simulink model "SistemSortareBandaTransportoare"  (R2025b)
settings: Solver=ode45  StartTime=0.0  StopTime=60  MaxStep=0.01  RelTol=1e-3
libraries: slpidlib x1
settings Model: Creator=Carina  LastModifiedBy=Carina

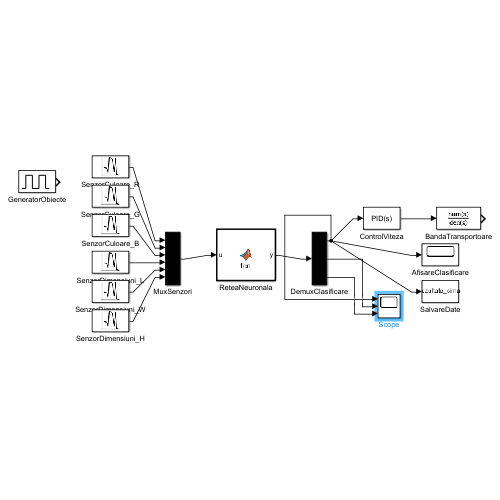
[thumbnail: Simulink's stored preview of the top-level diagram]
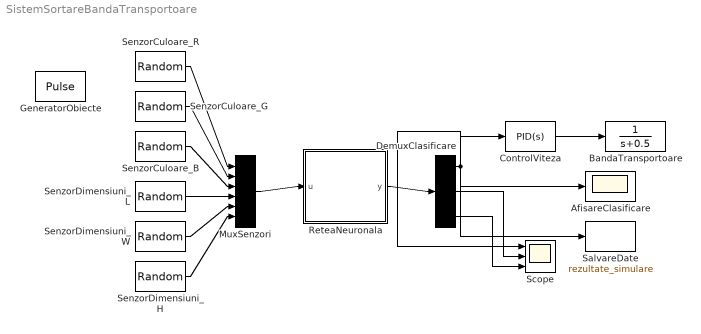
== system SistemSortareBandaTransportoare ==
  AfisareClasificare : Scope
      settings: ActiveDisplayYMinimum=-0.36488795691519493  ActiveDisplayYMaximum=1.6245350457686565
  BandaTransportoare : TransferFcn  Denominator=[1 0.5]
  ControlViteza : slpidlib/PID Controller  Controller=PID  Form=Parallel  TimeDomain=Continuous-time  UseExternalTs=off  SampleTime=-1  IntegratorMethod=Forward Euler  FilterMethod=Forward Euler  ControllerParametersSource=internal  P=1  I=1  UseKiTs=off  D=0  UseExternalDerivativeSource=off  N=100  UseFilter=on  TunerSelectOption=Transfer Function Based (PID Tuner App)  InitialConditionSource=internal  InitialConditionForIntegrator=0  InitialConditionForFilter=0  DifferentiatorICPrevScaledInput=0  ExternalReset=none  TrackingMode=off  Kt=1  LimitOutput=off  SatLimitsSource=internal  UpperSaturationLimit=inf  LowerSaturationLimit=-inf  LinearizeAsGain=on  AntiWindupMode=none  Kb=1  LimitIntegrator=off  UpperIntegratorSaturationLimit=inf  LowerIntegratorSaturationLimit=-inf  POutMin=[]  POutMax=[]  IOutMin=[]  IOutMax=[]  DOutMin=[]  DOutMax=[]  NOutMin=[]  NOutMax=[]  SumOutMin=[]  SumOutMax=[]  SaturationOutMin=[]  SaturationOutMax=[]  PParamMin=[]  PParamMax=[]  IParamMin=[]  IParamMax=[]  DParamMin=[]  DParamMax=[]  NParamMin=[]  NParamMax=[]  KbParamMin=[]  KbParamMax=[]  KtParamMin=[]  KtParamMax=[]  KbOutMin=[]  KbOutMax=[]  KtOutMin=[]  KtOutMax=[]  IntegratorOutMin=[]  IntegratorOutMax=[]  FilterOutMin=[]  FilterOutMax=[]  SumI1OutMin=[]  SumI1OutMax=[]  SumI2OutMin=[]  SumI2OutMax=[]  SumI3OutMin=[]  SumI3OutMax=[]  SumI4OutMin=[]  SumI4OutMax=[]  SumDOutMin=[]  SumDOutMax=[]  DifferentiatorOutMin=[]  DifferentiatorOutMax=[]  FilterDiffOutCoefMin=[]  FilterDiffOutCoefMax=[]  ReciprocalOutMin=[]  ReciprocalOutMax=[]  SumDenOutMin=[]  SumDenOutMax=[]  SumNumOutMin=[]  SumNumOutMax=[]  DivideOutMin=[]  DivideOutMax=[]  UdiffTsProdOutMin=[]  UdiffTsProdOutMax=[]  NTsProdOutMin=[]  NTsProdOutMax=[]  UintegralTsProdOutMin=[]  UintegralTsProdOutMax=[]  UngainTsProdOutMin=[]  UngainTsProdOutMax=[]  ClampingZeroOutDataTypeStr=Inherit: Inherit via back propagation  ClampingZeroOutMin=[]  ClampingZeroOutMax=[]  FilterDenConstantOutDataTypeStr=Inherit: Inherit via back propagation  FilterDenConstantOutMin=[]  FilterDenConstantOutMax=[]  PCopyOutDataTypeStr=Inherit: Inherit via back propagation  PCopyOutMin=[]  PCopyOutMax=[]  NCopyOutDataTypeStr=Inherit: Inherit via back propagation  NCopyOutMin=[]  NCopyOutMax=[]  IntegratorContinuousStateAttributes=''  IntegratorStateMustResolveToSignalObject=off  IntegratorRTWStateStorageClass=Auto  FilterContinuousStateAttributes=''  FilterStateMustResolveToSignalObject=off  FilterRTWStateStorageClass=Auto  ParallelPVariant=InternalParameters  IdealPVariant=Disabled  IVariant=InternalParameters  DVariant=InternalParameters  IntegratorVariant=Continuous  SatVariant=Disabled  AWVariant=Passthrough  PCopyVariant=Disabled  TRVariant=Disabled  FdbkBlocksVariant=Forward  IdealPFdbkVariant=Disabled  SatFdbkVariant=Disabled  DerivativeFilterVariant=ContFilter  NVariant=InternalParameters  NCopyVariant=Disabled  FilterICVariant=InternalICsFilter  IntegratorICVariant=InternalICs  ExternalResetVariant=Disabled  TRSumVariant=Passthrough  SumFdbkVariant=Disabled  SumVariant=Sum_PID  TsampFilterVariant=InternalTs  TsampNgainVariant=Passthrough  TsampIntegralVariant=Disabled_SignalSpec  ExternalSaturationOutDataTypeStr=Inherit: Same as second input  DerivativeSourceVariant=ErrorSignal  PreIntVariant=InternalPreInt
  DemuxClasificare : Demux  Outputs=3
  GeneratorObiecte : DiscretePulseGenerator  PulseType=Time based  PulseWidth=50
  MuxSenzori : Mux  Inputs=6
  ReteaNeuronala : MATLAB Function  TreatAsAtomicUnit=on
  SalvareDate : ToWorkspace  VariableName=rezultate_simulare  SaveFormat=Timeseries  SampleTime=-1
  Scope : Scope  NumInputPorts=3
      settings: ActiveDisplayYMinimum=-0.8870164568392116  ActiveDisplayYMaximum=1.6800836415005935
  SenzorCuloare_B : RandomNumber  Mean=128  Variance=50  SampleTime=0.1
  SenzorCuloare_G : RandomNumber  Mean=128  Variance=50  SampleTime=0.1
  SenzorCuloare_R : RandomNumber  Mean=128  Variance=50  SampleTime=0.1
  SenzorDimensiuni_H : RandomNumber  Mean=0.10  Variance=0.03  SampleTime=0.1
  SenzorDimensiuni_L : RandomNumber  Mean=0.15  Variance=0.05  SampleTime=0.1
  SenzorDimensiuni_W : RandomNumber  Mean=0.15  Variance=0.05  SampleTime=0.1
  wires:
  SenzorCuloare_R/1 -> MuxSenzori/1
  SenzorCuloare_G/1 -> MuxSenzori/2
  SenzorCuloare_B/1 -> MuxSenzori/3
  SenzorDimensiuni_L/1 -> MuxSenzori/4
  SenzorDimensiuni_W/1 -> MuxSenzori/5
  SenzorDimensiuni_H/1 -> MuxSenzori/6
  MuxSenzori/1 -> ReteaNeuronala/1(u)
  ReteaNeuronala/1(y) -> DemuxClasificare/1
  DemuxClasificare/1 -> Scope/1, SalvareDate/1, ControlViteza/1, AfisareClasificare/1
  ControlViteza/1 -> BandaTransportoare/1
  DemuxClasificare/2 -> Scope/2
  DemuxClasificare/3 -> Scope/3

== matlab function SistemSortareBandaTransportoare/ReteaNeuronala ==
  data: u input; y output
function y = fcn(u)
% u = [R G B L W H] (senzorii)
% y = [Plastic; Metal; Sticla] (vector cu 3 ieșiri)

% Normalizare manuală simplă
R = u(1)/255;
G = u(2)/255;
B = u(3)/255;
L = u(4)/0.3;
W = u(5)/0.3;
H = u(6)/0.3;

% Exemplu pseudo-clasificare (logică demo)
plastic_score = 1.5 - abs(R-0.5)*0.5 - L*0.2 - W*0.2;
metal_score   = (R+G+B)/3 + (L+W+H)*0.1;
sticla_score  = 1 - abs(G-0.6)*0.4 + H*0.2;

scores = [plastic_score, metal_score, sticla_score];

% Softmax, întotdeauna vector-coloană
exps = exp(scores - max(scores));
y = (exps ./ sum(exps))';     
y = y(:);
end
